simulink model "BLDCmotor_FOC_R2017b_fixdt"  (R2025a)
settings: Solver=FixedStepDiscrete  StartTime=0  StopTime=0.5  FixedStep=Ts  MaxStep=1e-6  RelTol=1e-6  AbsTol=1e-6  EnableMultiTasking=on
PreLoadFcn:
  | addpath(pwd);
  | addpath(genpath('01_Libraries'));
  | addpath(genpath('02_Figures'));
  | addpath(genpath('03_CreateParamTable'));
InitFcn:
  | init_model;
values from neighbouring files (symbols this model uses):
  a_cpr = 65535    [init_model.m]
  a_elecAngle = 60    [init_model.m]
  a_elecoffset = a_elecPeriod/12    (= 30)    [init_model.m]
  a_elecPeriod = 360    [init_model.m]
  a_fcpr = 1/65535    (= 1.52590218967e-05)    [init_model.m]
  a_mechoffset = a_elecoffset/n_polePairs    (= 5)    [init_model.m]
  a_phaAdvMax = 25    [init_model.m]
  b_angleMeasEna = 1    [init_model.m]
  b_cruiseCtrlEna = 0    [init_model.m]
  b_diagEna = 0    [init_model.m]
  b_fieldWeakEna = 0    [init_model.m]
  cf_currFilt = 0.692    [init_model.m]
  cf_idKi = Ki / (f_ctrl)    (= 0.00409061543436)    [init_model.m]
  cf_idKp = Kp    (= 0.0523598775598)    [init_model.m]
  cf_iqKi = Ki / (f_ctrl)    (= 0.00409061543436)    [init_model.m]
  cf_iqKiLimProt = 60 / (f_ctrl)    (= 0.00375)    [init_model.m]
  cf_iqKp = Kp    (= 0.0523598775598)    [init_model.m]
  cf_KbLimProt = Simulink.Parameter    [init_model.m]
  cf_nKi = 20.4 / (f_ctrl)    (= 0.001275)    [init_model.m]
  cf_nKiLimProt = 20 / (f_ctrl)    (= 0.00125)    [init_model.m]
  cf_nKp = 1.18    [init_model.m]
  cf_speedCoef = round(f_ctrl * a_mechAngle * (pi/180) * (30/pi))    [init_model.m]
  CTRL_FOC = 2    [init_model.m]
  CTRL_SIN = 1    [init_model.m]
  dV_openRate = 1000 / (f_ctrl)    (= 0.0625)    [init_model.m]
  dz_cntTrnsDetHi = 40    [init_model.m]
  dz_cntTrnsDetLo = 20    [init_model.m]
  ff_gain = ((r_motn / i_sca) * ((GD32_Vd_max_margin) / v_bus))    (= 0.338958333333)    [init_model.m]
  GD32_Vd_max_margin = GD32_Vd_max - V_margin    (= 1627)    [init_model.m]
  GD32_Vq_max_M1 = sqrt(GD32_Vd_max_margin^2 - GD32_Vq_max_XA.^2)    [init_model.m]
  i_max = i_max * i_sca    (= 500)    [init_model.m]
  id_fieldWeakMax = 5 * i_sca    (= 250)    [init_model.m]
  iq_maxSca_M1 = sqrt(1 - iq_maxSca_XA.^2)    [init_model.m]
  mcu_model = GD32F103    (= 1)    [init_model.m]
  n_commAcvLo = 15    [init_model.m]
  n_commDeacvHi = 30    [init_model.m]
  n_cruiseMotTgt = 0    [init_model.m]
  n_fieldWeakAuthHi = 300    [init_model.m]
  n_fieldWeakAuthLo = 100    [init_model.m]
  n_max = 1950    [init_model.m]
  n_polePairs = 6    [init_model.m]
  n_stdStillDet = 3    [init_model.m]
  OPEN_MODE = 0    [init_model.m]
  r_cos_M1 = cos((a_elecAngle_XA + a_elecPeriod/12)*(pi/180))    [init_model.m]
  r_errInpTgtThres = 600    [init_model.m]
  r_fieldWeakHi = 1000    [init_model.m]
  r_fieldWeakLo = 750    [init_model.m]
  r_motn = r_mot/2    (= 0.25)    [init_model.m]
  r_sin3PhaA_M1 = sin3Arm + A*r_sinPhaA_M1    [init_model.m]
  r_sin3PhaB_M1 = sin3Arm + A*r_sinPhaB_M1    [init_model.m]
  r_sin3PhaC_M1 = sin3Arm + A*r_sinPhaC_M1    [init_model.m]
  r_sin_M1 = sin((a_elecAngle_XA + a_elecPeriod/12)*(pi/180))    [init_model.m]
  SPD_MODE = 2    [init_model.m]
  STM32_Vd_max_margin = STM32_Vd_max - V_margin    (= 940)    [init_model.m]
  STM32_Vq_max_M1 = sqrt(STM32_Vd_max_margin^2 - STM32_Vq_max_XA.^2)    [init_model.m]
  t_errDequal = 1.80 * f_ctrl    (= 28800)    [init_model.m]
  t_errQual = 0.24 * f_ctrl    (= 3840)    [init_model.m]
  tgt_scale = 2047    [init_model.m]
  TRQ_MODE = 3    [init_model.m]
  Ts = 5e-6    (= 5e-06)    [init_model.m]
  Ts_ctrl = 6e-5    (= 6e-05)    [init_model.m]
  v_bus = 24    [init_model.m]
  vec_hallToPos = [0 2 0 1 4 3 5 0]    [init_model.m]
  VLT_MODE = 1    [init_model.m]
  z_commutMap_M1 = [-1 -1  0  1  1  0 ... (first row only)    [init_model.m]
  z_ctrlModReq = TRQ_MODE    (= 3)    [init_model.m]
  z_ctrlTypSel = CTRL_FOC    (= 2)    [init_model.m]
  z_maxCntRst = 2000    [init_model.m]
  z_selPhaCurMeasABC = 2    [init_model.m]
undefined symbols (not defined in the file or in its folder): BLDCmotor_FOC_R2017b_fixdt, DiscIntNeverNeededParam, DWORK0, DWORK1, DWORK2, DWORK3, powergui, spspowerguiLib
libraries: BLDC_controller_Lib x18, simulink x13, prociolib x6, eePwmGenerator x6, eePwmGeneratorMultilevel x3, mcbpositiondecoderlib x2, slpidlib x2, spsControlledVoltageSourceLib x1, spsMultimeterLib x1, spsPermanentMagnetSynchronousMachineLib x1, spsUniversalBridgeLib x1, spsVoltageMeasurementLib x1
(part 2 of 6)

== system BLDCmotor_FOC_R2017b_fixdt/PWM_gates ==
  DC_pha : Inport
  Abs : Abs  Commented=on  OutDataTypeStr=Inherit: Inherit via back propagation  RndMeth=Zero  SaturateOnIntegerOverflow=off
  Abs1 : Abs  Commented=on  OutDataTypeStr=Inherit: Inherit via back propagation  RndMeth=Zero  SaturateOnIntegerOverflow=off
  Abs2 : Abs  Commented=on  OutDataTypeStr=Inherit: Inherit via back propagation  RndMeth=Zero  SaturateOnIntegerOverflow=off
  Constant3 : Constant  Commented=on  Value=0  OutDataTypeStr=Inherit: Inherit via back propagation
  Constant4 : Constant  Commented=on  OutDataTypeStr=Inherit: Inherit via back propagation
  Demux : Demux  Commented=on  Outputs=3
  Demux1 : Demux  Commented=on  Outputs=3
  MCU_VD_Selector : Subsystem  Commented=on
  MinMax : MinMax  Commented=on  Inputs=2  OutDataTypeStr=Inherit: Inherit via back propagation  RndMeth=Zero
  MinMax1 : MinMax  Commented=on  Function=max  Inputs=2  OutDataTypeStr=Inherit: Inherit via back propagation  RndMeth=Zero
  MinMax2 : MinMax  Commented=on  Inputs=2  OutDataTypeStr=Inherit: Inherit via back propagation  RndMeth=Zero
  MinMax3 : MinMax  Commented=on  Function=max  Inputs=2  OutDataTypeStr=Inherit: Inherit via back propagation  RndMeth=Zero
  MinMax4 : MinMax  Commented=on  Inputs=2  OutDataTypeStr=Inherit: Inherit via back propagation  RndMeth=Zero
  MinMax5 : MinMax  Commented=on  Function=max  Inputs=2  OutDataTypeStr=Inherit: Inherit via back propagation  RndMeth=Zero
  Mux1 : Mux  Commented=on  Inputs=6
  Mux4 : Mux  Commented=on  Inputs=3
  "PWM Gate Signal Generator (Three-phase, Two-level)" : eePwmGeneratorTwoLevel/PWM Gate Signal Generator (Three-phase, Two-level)  Commented=on  fsw=1e3  Ts=5e-5
      settings: SamplingMode=Natural
      settings: LibrarySourceBlock=|
      | ee_sl_lib/Pulse Width
      | Modulation/PWM Gate Signal Generator
      | (Three-phase, Two-level)
  PWM Generator (2-Level) : spsPWMGenerator2LevelLib/PWM Generator (2-Level)  ModulatorType=Three-phase bridge (6 pulses)  ModulatorMode=Unsynchronized  Fc=16000  Pc=90  nF=27  MinMax=[-1627 1627]  SamplingTechnique=Natural  ModulatingSignals=off  m=0.8  Freq=60  Phase=0  Ts=Ts  ShowCarrierOutport=on
  PWM Generator (Multilevel) : eePwmGeneratorMultilevel/PWM Generator (Multilevel)  Commented=on  topology=Half-bridge  Nsm=1  Tper=6.25e-5  Ts=5e-6
      settings: LibrarySourceBlock=|
      | ee_sl_lib/Pulse Width
      | Modulation/PWM Generator
      | (Multilevel)
  PWM Generator (Multilevel)1 : eePwmGeneratorMultilevel/PWM Generator (Multilevel)  Commented=on  topology=Half-bridge  Nsm=1  Tper=6.25e-5  Ts=5e-6
      settings: LibrarySourceBlock=|
      | ee_sl_lib/Pulse Width
      | Modulation/PWM Generator
      | (Multilevel)
  PWM Generator (Multilevel)2 : eePwmGeneratorMultilevel/PWM Generator (Multilevel)  Commented=on  topology=Half-bridge  Nsm=1  Tper=6.25e-5  Ts=5e-6
      settings: LibrarySourceBlock=|
      | ee_sl_lib/Pulse Width
      | Modulation/PWM Generator
      | (Multilevel)
  PWM Write : prociolib/PWM Write  Commented=on  ShowPeriodInp=off  ShowPhaseInp=off  PeripheralConfigBtnCtrl=0  BlockSID=BLDCmotor_FOC_R2017b_fixdt:22845
  PWM Write1 : prociolib/PWM Write  Commented=on  ShowPeriodInp=off  ShowPhaseInp=off  PeripheralConfigBtnCtrl=0  BlockSID=BLDCmotor_FOC_R2017b_fixdt:22846
  PWM Write2 : prociolib/PWM Write  Commented=on  ShowPeriodInp=off  ShowPhaseInp=off  PeripheralConfigBtnCtrl=0  BlockSID=BLDCmotor_FOC_R2017b_fixdt:22847
  PWM Write3 : prociolib/PWM Write  Commented=on  ShowPeriodInp=off  ShowPhaseInp=off  PeripheralConfigBtnCtrl=0  BlockSID=BLDCmotor_FOC_R2017b_fixdt:22848
  PWM Write4 : prociolib/PWM Write  Commented=on  ShowPeriodInp=off  ShowPhaseInp=off  PeripheralConfigBtnCtrl=0  BlockSID=BLDCmotor_FOC_R2017b_fixdt:22849
  PWM Write5 : prociolib/PWM Write  Commented=on  ShowPeriodInp=off  ShowPhaseInp=off  PeripheralConfigBtnCtrl=0  BlockSID=BLDCmotor_FOC_R2017b_fixdt:22850
  PWM_generator{,6..10} (6 alike) : eePwmGenerator/PWM Generator  Commented=on  CarrCount=Up  Tper=5e-05  Tdelay=0  Ts=Ts
  PWM_generator1 : Subsystem  Commented=on
      mask help: Simulink:masks:GenSFuncDesc_MD
      mask Help: eval('feval(''rtwprivate'',''rtwhelpview'',''rtw_sfcn_block'')');
  PWM_generator12 : Subsystem  Commented=on
      mask help: Simulink:masks:GenSFuncDesc_MD
      mask Help: eval('feval(''rtwprivate'',''rtwhelpview'',''rtw_sfcn_block'')');
  PWM_generator2 : Subsystem  Commented=on
      mask help: Simulink:masks:GenSFuncDesc_MD
      mask Help: eval('feval(''rtwprivate'',''rtwhelpview'',''rtw_sfcn_block'')');
  PWM_generator3 : Subsystem  Commented=on
      mask help: Simulink:masks:GenSFuncDesc_MD
      mask Help: eval('feval(''rtwprivate'',''rtwhelpview'',''rtw_sfcn_block'')');
  PWM_generator4 : Subsystem  Commented=on
      mask help: Simulink:masks:GenSFuncDesc_MD
      mask Help: eval('feval(''rtwprivate'',''rtwhelpview'',''rtw_sfcn_block'')');
  PWM_generator5 : Subsystem  Commented=on
      mask help: Simulink:masks:GenSFuncDesc_MD
      mask Help: eval('feval(''rtwprivate'',''rtwhelpview'',''rtw_sfcn_block'')');
  Terminator : Terminator
  Vd_max2 : Constant  Commented=on  Value=mcu_model  OutDataTypeStr=boolean
  signal_log6 : Subsystem  Commented=on
  gates_PWM : Outport  VectorParamsAs1DForOutWhenUnconnected=off
  wires:
  MCU_VD_Selector/1(Out1) -> ?
  Vd_max2/1 -> MCU_VD_Selector/1(In1)
  PWM Generator (Multilevel)1/1 -> Mux4/2
  Demux/3 -> PWM Generator (Multilevel)2/1
  Demux/2 -> PWM Generator (Multilevel)1/1
  ? -> Demux/1
  PWM Generator (Multilevel)/1 -> Mux4/1
  Demux/1 -> PWM Generator (Multilevel)/1
  PWM Generator (Multilevel)2/1 -> Mux4/3
  Abs2/1 -> PWM_generator10/1
  MinMax3/1 -> PWM_generator7/1
  PWM_generator8/1 -> Mux1/4
  MinMax5/1 -> PWM_generator9/1
  Abs1/1 -> PWM_generator8/1
  MinMax2/1 -> Abs1/1
  MinMax4/1 -> Abs2/1
  Abs/1 -> PWM_generator6/1
  PWM_generator6/1 -> Mux1/2
  Demux1/1 -> MinMax/2, MinMax1/2
  PWM_generator7/1 -> Mux1/3
  MinMax/1 -> Abs/1
  Demux1/2 -> MinMax2/2, MinMax3/2
  PWM_generator/1 -> Mux1/1
  PWM_generator9/1 -> Mux1/5
  Constant4/1 -> MinMax5/1, MinMax3/1, MinMax1/1
  MinMax1/1 -> PWM_generator/1
  PWM_generator10/1 -> Mux1/6
  Demux1/3 -> MinMax5/2, MinMax4/2
  Constant3/1 -> MinMax4/1, MinMax2/1, MinMax/1
  ? -> Demux1/1
  DC_pha/1 -> PWM Generator (2-Level)/1
  PWM Generator (2-Level)/1 -> gates_PWM/1
  PWM Generator (2-Level)/2 -> Terminator/1

== system BLDCmotor_FOC_R2017b_fixdt/Power Stage ==
  DC_pha : Inport
  LdTrq : Inport  Port=2
  Bus Creator : BusCreator  Inputs=4
  Bus Creator1 : BusCreator  Inputs=13
  Bus Selector : BusSelector  OutputSignals=signal1.IaStator,signal1.IbStator,signal1.IcStator,signal1.IqSync,signal1.IdSync,signal1.VqSync,signal1.VdSync,Hall.signal1,Hall.signal2,Hall.signal3  OutputAsBus=on
  Bus Selector1 : BusSelector  OutputSignals=signal1.MtrSpd,signal1.MtrPos,signal1.MtrTrq  OutputAsBus=on
  Bus Selector3 : BusSelector  OutputSignals=MtrElcPos  OutputAsBus=on
  Constant1 : Constant  Value=v_bus
  Data Type Conversion9 : DataTypeConversion  OutDataTypeStr=double  SaturateOnIntegerOverflow=off
  Demux1 : Demux  Outputs=[1,1,1,1,1,1,1,1,1,1]
  Demux2 : Demux  Outputs=[1,1,1]
  Divide : Product  Inputs=*/
  Product : Product
  Scope : Scope  NumInputPorts=3
      settings: ActiveDisplayYMinimum=-159.83844430308204  ActiveDisplayYMaximum=171.67027137436321  DataLoggingVariableName=ScopeData12
  Subsystem : Subsystem
  Surface Mount PMSM : autolibpmsmexterior/Surface Mount PMSM  port_config=Torque  sim_type=Discrete  Ts=5e-06  P=n_polePairs  Rs=r_motn  Ldq_=L_ph  KConstText=Torque constant (Kt):  lambda_pm=0.2205  Ke=160  Kt=1  mechanical=[0.0027, 0.1, 0]  idq0=[0 0]  theta_init=0  omega_init=0  KConst=0.2205  lambda_pm_calc=0.2205  RefBlkName='autolibpmsmexterior/Surface Mount PMSM'  aMode=5  Ldq="[0.0017      0.0017]"
  Variant Subsystem : Subsystem  Variant=on  VariantActivationTime=code compile
  motor_out : Outport  VectorParamsAs1DForOutWhenUnconnected=off
  wires:
  Data Type Conversion9/1 -> Divide/2
  Variant Subsystem/1(Vd_max_margin) -> Data Type Conversion9/1
  DC_pha/1 -> Scope/3, Product/2
  Product/1 -> Scope/2, Surface Mount PMSM/2
  Surface Mount PMSM/2 -> Bus Creator/2
  Surface Mount PMSM/3 -> Bus Creator/3
  LdTrq/1 -> Surface Mount PMSM/1
  Bus Creator/1 -> Bus Selector/1, Bus Selector1/1
  Bus Creator1/1 -> motor_out/1  "<IcStator>"
  Bus Selector3/1 -> Subsystem/1(the)
  Surface Mount PMSM/1 -> Bus Selector3/1, Bus Creator/1
  Demux1/1 -> Bus Creator1/1  "Stator current is_a (A)"
  Demux1/8 -> Bus Creator1/8  "Hall effect signal h_a"
  Demux1/10 -> Bus Creator1/10  "Hall effect signal h_c"
  Demux2/1 -> Bus Creator1/11  "Rotor speed wm (rad/s)"
  Demux2/3 -> Bus Creator1/13  "Electromagnetic torque Te (N*m)"
  Demux1/6 -> Bus Creator1/6  "Stator voltage Vs_q (V)"
  Demux1/9 -> Bus Creator1/9  "Hall effect signal h_b"
  Demux1/2 -> Bus Creator1/2  "Stator current is_b (A)"
  Demux1/5 -> Bus Creator1/5  "Stator current is_d (A)"
  Demux1/4 -> Bus Creator1/4  "Stator current is_q (A)"
  Demux1/7 -> Bus Creator1/7  "Stator voltage Vs_d (V)"
  Demux1/3 -> Bus Creator1/3  "Stator current is_c (A)"
  Demux2/2 -> Bus Creator1/12  "Rotor angle thetam (rad)"
  Subsystem/1(Hall) -> Bus Creator/4  "Hall"
  Bus Selector/1 -> Demux1/1
  Bus Selector1/1 -> Demux2/1
  Constant1/1 -> Divide/1
  Divide/1 -> Scope/1, Product/1

== system BLDCmotor_FOC_R2017b_fixdt/Theoretical_Speed_Trajectory ==
  note: Ideal Speed Trajectory Calculation
      | Based on Min/Max torque and Min/Max torque rate constraints
  r_inpTgtRaw : Inport
  Discrete Derivative1 : simulink/Discrete/Discrete Derivative  gainval=1.0  ICPrevScaledInput=0.0  OutMin=[]  OutMax=[]  OutDataType=fixdt(1, 16)  OutScaling=2^-10  DoSatur=off
  Discrete Derivative2 : simulink/Discrete/Discrete Derivative  gainval=1.0  ICPrevScaledInput=0.0  OutMin=[]  OutMax=[]  OutDataType=fixdt(1, 16)  OutScaling=2^-10  DoSatur=off
  Discrete-Time Integrator2 : DiscreteIntegrator  SampleTime=-1  ICPrevOutput=DiscIntNeverNeededParam  ICPrevScaledInput=DiscIntNeverNeededParam
  Divide2 : Product  Inputs=*/
  Divide3 : Product  Inputs=**
  Divide4 : Product  Inputs=**
  Gain1 : Gain  Gain=-1
  Gain2 : Gain  Gain=-1
  Gain4 : Gain  Gain=pi/30
  Gain5 : Gain  Gain=30/pi
  J_mot : Constant  Value=0.01  OutDataTypeStr=Inherit: Inherit via back propagation
  Kp : Constant  Value=65  OutDataTypeStr=Inherit: Inherit via back propagation
  M_max : Constant  Value=15  OutDataTypeStr=Inherit: Inherit via back propagation
  Manual Switch : ManualSwitch
  Mux4 : Mux  Inputs=2
  Rate Limiter Dynamic3 : simulink/Discontinuities/Rate Limiter Dynamic
  Saturation Dynamic : simulink/Discontinuities/Saturation Dynamic  OutMin=[]  OutMax=[]  OutDataTypeStr=Inherit: Same as second input  OutDataType=fixdt(1, 16)  OutScaling=2^-10  DoSatur=off
  Scope : Scope  NumInputPorts=3
      settings: ActiveDisplayYMinimum=-1250  ActiveDisplayYMaximum=1250
  Sum2 : Sum  Inputs=|+-  RndMeth=Zero  OutDataTypeStr=Inherit: Same as first input
  Sum8 : Sum  Inputs=++|  RndMeth=Zero  OutDataTypeStr=Inherit: Same as first input
  dM_max : Constant  Value=500  OutDataTypeStr=Inherit: Inherit via back propagation
  r_inpTgt : Outport  VectorParamsAs1DForOutWhenUnconnected=off
  wires:
  Gain4/1 -> Divide4/2  "dw"
  M_max/1 -> Gain1/1, Saturation Dynamic/1
  J_mot/1 -> Divide2/2, Divide4/1
  Divide2/1 -> Gain5/1  "w"
  [r_inpTgtRaw] -> Discrete Derivative2/1, Sum2/1
  Divide4/1 -> Saturation Dynamic/2  "M"
  Gain1/1 -> Saturation Dynamic/3
  dM_max/1 -> Gain2/1, Rate Limiter Dynamic3/1
  Sum2/1 -> Divide3/2
  Divide3/1 -> Sum8/2
  Rate Limiter Dynamic3/1 -> [M_tgtTheo], Discrete-Time Integrator2/1
  Gain2/1 -> Rate Limiter Dynamic3/3
  Sum8/1 -> Gain4/1  "dn"
  Saturation Dynamic/1 -> Rate Limiter Dynamic3/2
  Gain5/1 -> [r_inpTgt], Sum2/2  "rpm"
  Kp/1 -> Divide3/1
  Discrete-Time Integrator2/1 -> Divide2/1
  Mux4/1 -> Scope/1
  Discrete Derivative1/1 -> Scope/3
  Discrete Derivative2/1 -> Sum8/1
  [M_tgtTheo] -> Discrete Derivative1/1, Scope/2
  r_inpTgtRaw/1 -> [r_inpTgtRaw]
  [r_inpTgtRaw] -> Mux4/1
  [r_inpTgt] -> Mux4/2
  [r_inpTgt] -> Manual Switch/2
  Manual Switch/1 -> r_inpTgt/1
  [r_inpTgtRaw] -> Manual Switch/1

== system BLDCmotor_FOC_R2017b_fixdt/filtLowPass ==
  u : Inport
  coef : Inport  Port=2
  Data Type Conversion23 : DataTypeConversion  OutDataTypeStr=fixdt(1,32,6)  SaturateOnIntegerOverflow=off  RndMeth=Floor
  Low_Pass_Filter : Subsystem
      settings: RTWFcnNameOpts=Use subsystem name
      mask Display:
      | plot(0,0,100,100, ...
      | [73,75,73,75,25,25,28,25,22,25],[18,20,22,20,20,84,82,84,82,84], ...
      | [25,33,33,72],[20,20,70,70],[33,34,36,39,44,50,56,66,73],[20,25,33,43,55,63,66,70,70]);
      | text(50,40,'coef'),
  y : Outport  VectorParamsAs1DForOutWhenUnconnected=off
  wires:
  coef/1 -> Low_Pass_Filter/2(coef)
  Low_Pass_Filter/1(y) -> y/1
  u/1 -> Data Type Conversion23/1
  Data Type Conversion23/1 -> Low_Pass_Filter/1(u)

== system BLDCmotor_FOC_R2017b_fixdt/mixer ==
  speed : Inport
  steer : Inport  Port=2
  speed_coef : Inport  Port=3
  steer_coef : Inport  Port=4
  Data Type Conversion2 : DataTypeConversion  OutDataTypeStr=int16  SaturateOnIntegerOverflow=off  RndMeth=Floor
  Data Type Conversion3 : DataTypeConversion  OutDataTypeStr=int16  SaturateOnIntegerOverflow=off  RndMeth=Floor
  Data Type Conversion4 : DataTypeConversion  OutDataTypeStr=int16  SaturateOnIntegerOverflow=off  RndMeth=Floor
  Display : Display
  Display1 : Display
  Display3 : Display
  Divide1 : Product  Inputs=**  RndMeth=Simplest  OutDataTypeStr=Inherit: Same as first input
  Divide2 : Product  Inputs=**  RndMeth=Simplest  OutDataTypeStr=Inherit: Same as first input
  Sum1 : Sum  Inputs=+-  InputSameDT=on  RndMeth=Simplest  SaturateOnIntegerOverflow=on  OutDataTypeStr=Inherit: Same as first input
  Sum2 : Sum  InputSameDT=on  RndMeth=Simplest  SaturateOnIntegerOverflow=on  OutDataTypeStr=Inherit: Same as first input
  speedR : Outport  VectorParamsAs1DForOutWhenUnconnected=off
  speedL : Outport  Port=2  VectorParamsAs1DForOutWhenUnconnected=off
  wires:
  Sum1/1 -> Data Type Conversion2/1
  speed/1 -> [speed]
  steer/1 -> [steer]
  speed_coef/1 -> [speed_coef]
  steer_coef/1 -> [steer_coef]
  [speed] -> Divide1/1
  [speed_coef] -> Divide1/2
  [steer] -> Divide2/1
  [steer_coef] -> Divide2/2
  Divide1/1 -> Display1/1, Data Type Conversion4/1, Sum2/1, Sum1/1
  Divide2/1 -> Sum2/2, Sum1/2
  Data Type Conversion2/1 -> speedR/1
  Data Type Conversion3/1 -> speedL/1
  Data Type Conversion4/1 -> Display/1
  Sum2/1 -> Display3/1, Data Type Conversion3/1

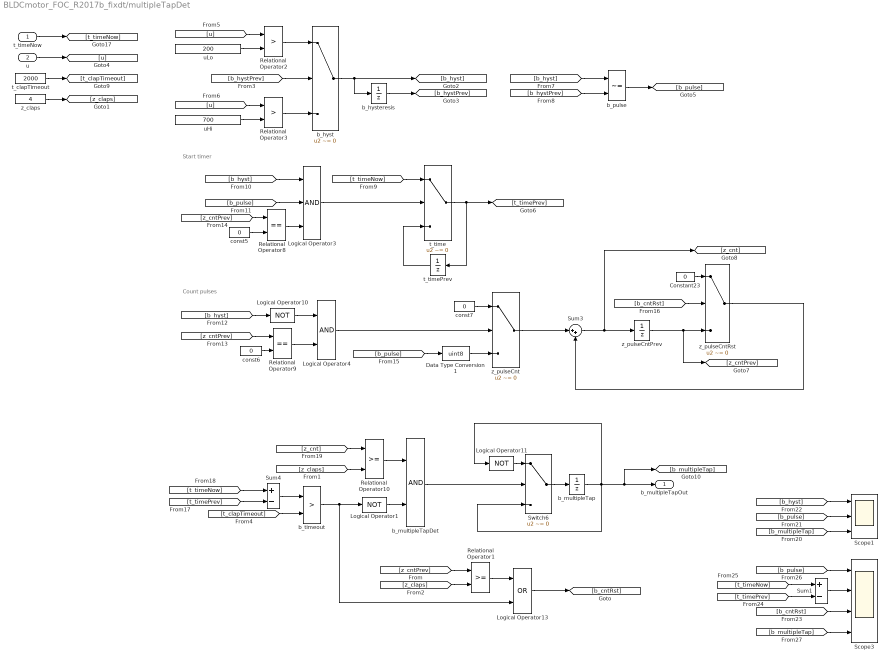
== system BLDCmotor_FOC_R2017b_fixdt/multipleTapDet ==
  note: Count pulses
  note: Start timer
  t_timeNow : Inport
  u : Inport  Port=2
  Constant23 : Constant  Value=0  OutDataTypeStr=Inherit: Inherit via back propagation
  Data Type Conversion1 : DataTypeConversion  OutDataTypeStr=uint8  SaturateOnIntegerOverflow=off  RndMeth=Floor
  Logical Operator1 : Logic  Operator=NOT  AllPortsSameDT=off  OutDataTypeStr=boolean
  Logical Operator10 : Logic  Operator=NOT  AllPortsSameDT=off  OutDataTypeStr=boolean
  Logical Operator11 : Logic  Operator=NOT  AllPortsSameDT=off  OutDataTypeStr=boolean
  Logical Operator13 : Logic  Operator=OR  AllPortsSameDT=off  OutDataTypeStr=boolean
  Logical Operator3 : Logic  Inputs=3  AllPortsSameDT=off  OutDataTypeStr=boolean
  Logical Operator4 : Logic  AllPortsSameDT=off  OutDataTypeStr=boolean
  Relational Operator1 : RelationalOperator  OutDataTypeStr=boolean  RndMeth=Simplest  InputSameDT=off
  Relational Operator10 : RelationalOperator  OutDataTypeStr=boolean  RndMeth=Simplest  InputSameDT=off
  Relational Operator2 : RelationalOperator  Operator=>  OutDataTypeStr=boolean  RndMeth=Simplest  InputSameDT=off
  Relational Operator3 : RelationalOperator  Operator=>  OutDataTypeStr=boolean  RndMeth=Simplest  InputSameDT=off
  Relational Operator8 : RelationalOperator  Operator===  OutDataTypeStr=boolean  RndMeth=Simplest  InputSameDT=off
  Relational Operator9 : RelationalOperator  Operator===  OutDataTypeStr=boolean  RndMeth=Simplest  InputSameDT=off
  Scope1 : Scope  NumInputPorts=3
      settings: ActiveDisplayYMinimum=-0.125  ActiveDisplayYMaximum=1.125
  Scope3 : Scope  NumInputPorts=4
      settings: ActiveDisplayYMinimum=-0.125  ActiveDisplayYMaximum=1.125
  Sum1 : Sum  Inputs=+-
  Sum3 : Sum  Inputs=|++
  Sum4 : Sum  Inputs=+-
  Switch6 : Switch  Criteria=u2 ~= 0  OutDataTypeStr=Inherit: Inherit via back propagation  RndMeth=Zero  SaturateOnIntegerOverflow=off  InputSameDT=off
  b_hyst : Switch  Criteria=u2 ~= 0  RndMeth=Zero  SaturateOnIntegerOverflow=off  InputSameDT=off
  b_hysteresis : UnitDelay  SampleTime=-1  HasFrameUpgradeWarning=on
      settings: AttributesFormatString=Ini=%<X0>
  b_multipleTap : UnitDelay  SampleTime=-1  HasFrameUpgradeWarning=on
      settings: AttributesFormatString=Ini=%<X0>
  b_multipleTapDet : Logic  AllPortsSameDT=off  OutDataTypeStr=boolean
  b_pulse : RelationalOperator  Operator=~=  OutDataTypeStr=boolean  RndMeth=Simplest  InputSameDT=off
  b_timeout : RelationalOperator  Operator=>  OutDataTypeStr=boolean  RndMeth=Simplest  InputSameDT=off
  const5 : Constant  Value=0  OutDataTypeStr=Inherit: Inherit via back propagation
  const6 : Constant  Value=0  OutDataTypeStr=Inherit: Inherit via back propagation
  const7 : Constant  Value=0  OutDataTypeStr=Inherit: Inherit via back propagation
  t_clapTimeout : Constant  Value=2000  OutDataTypeStr=Inherit: Inherit via back propagation
  t_time : Switch  Criteria=u2 ~= 0  OutDataTypeStr=Inherit: Inherit via back propagation  RndMeth=Zero  SaturateOnIntegerOverflow=off  InputSameDT=off
  t_timePrev : UnitDelay  SampleTime=-1  HasFrameUpgradeWarning=on
      settings: AttributesFormatString=Ini=%<X0>
  uHi : Constant  Value=700  OutDataTypeStr=Inherit: Inherit via back propagation
  uLo : Constant  Value=200  OutDataTypeStr=Inherit: Inherit via back propagation
  z_claps : Constant  Value=4  OutDataTypeStr=Inherit: Inherit via back propagation
  z_pulseCnt : Switch  Criteria=u2 ~= 0  OutDataTypeStr=Inherit: Inherit via back propagation  RndMeth=Zero  SaturateOnIntegerOverflow=off  InputSameDT=off
  z_pulseCntPrev : UnitDelay  SampleTime=-1  HasFrameUpgradeWarning=on
      settings: AttributesFormatString=Ini=%<X0>
  z_pulseCntRst : Switch  Criteria=u2 ~= 0  OutDataTypeStr=Inherit: Inherit via back propagation  RndMeth=Simplest  SaturateOnIntegerOverflow=off  InputSameDT=off
  b_multipleTapOut : Outport  VectorParamsAs1DForOutWhenUnconnected=off
  wires:
  t_timeNow/1 -> [t_timeNow]
  Relational Operator2/1 -> b_hyst/1
  b_hyst/1 -> b_hysteresis/1, [b_hyst]
  uLo/1 -> Relational Operator2/2
  b_hysteresis/1 -> [b_hystPrev]
  [b_hystPrev] -> b_hyst/2
  uHi/1 -> Relational Operator3/2
  Relational Operator3/1 -> b_hyst/3
  u/1 -> [u]
  [u] -> Relational Operator2/1
  [u] -> Relational Operator3/1
  [b_hyst] -> b_pulse/1
  [b_hystPrev] -> b_pulse/2
  b_pulse/1 -> [b_pulse]
  t_time/1 -> t_timePrev/1, [t_timePrev]
  t_timePrev/1 -> t_time/3
  [t_timeNow] -> t_time/1
  const5/1 -> Relational Operator8/2
  Relational Operator8/1 -> Logical Operator3/3
  Logical Operator3/1 -> t_time/2
  [b_hyst] -> Logical Operator3/1
  [b_pulse] -> Logical Operator3/2
  Data Type Conversion1/1 -> z_pulseCnt/3
  const7/1 -> z_pulseCnt/1
  Logical Operator4/1 -> z_pulseCnt/2
  const6/1 -> Relational Operator9/2
  Relational Operator9/1 -> Logical Operator4/2
  Logical Operator10/1 -> Logical Operator4/1
  [b_pulse] -> Data Type Conversion1/1
  [b_hyst] -> Logical Operator10/1
  [z_cntPrev] -> Relational Operator9/1
  [z_cntPrev] -> Relational Operator8/1
  z_pulseCnt/1 -> Sum3/1
  Sum4/1 -> b_timeout/1
  [t_timePrev] -> Sum4/2
  [t_timeNow] -> Sum4/1
  [t_clapTimeout] -> b_timeout/2
  Logical Operator11/1 -> Switch6/1
  b_multipleTap/1 -> Switch6/3, [b_multipleTap], b_multipleTapOut/1, Logical Operator11/1
  Switch6/1 -> b_multipleTap/1
  [z_claps] -> Relational Operator10/2
  [z_cnt] -> Relational Operator10/1
  Relational Operator10/1 -> b_multipleTapDet/1
  b_timeout/1 -> Logical Operator13/2, Logical Operator1/1
  [b_pulse] -> Scope1/2
  [b_hyst] -> Scope1/1
  b_multipleTapDet/1 -> Switch6/2
  Logical Operator13/1 -> [b_cntRst]
  [z_cntPrev] -> Relational Operator1/1
  [z_claps] -> Relational Operator1/2
  Relational Operator1/1 -> Logical Operator13/1
  [b_cntRst] -> z_pulseCntRst/2
  Constant23/1 -> z_pulseCntRst/1
  z_pulseCntPrev/1 -> [z_cntPrev], z_pulseCntRst/3
  z_pulseCntRst/1 -> Sum3/2
  z_claps/1 -> [z_claps]
  t_clapTimeout/1 -> [t_clapTimeout]
  Logical Operator1/1 -> b_multipleTapDet/2
  Sum3/1 -> [z_cnt], z_pulseCntPrev/1
  [t_timeNow] -> Sum1/1
  [t_timePrev] -> Sum1/2
  [b_pulse] -> Scope3/1
  Sum1/1 -> Scope3/2
  [b_cntRst] -> Scope3/3
  [b_multipleTap] -> Scope1/3
  [b_multipleTap] -> Scope3/4

== system BLDCmotor_FOC_R2017b_fixdt/rad2deg ==
  note: Convert mechanical angle to electrical angle.
  rad : Inport
  Constant : Constant  Value=360
  Constant1 : Constant  Value=n_polePairs
  Divide : Product  Inputs=**
  Gain4 : Gain  Gain=180/pi  RndMeth=Zero  OutDataTypeStr=Inherit: Same as input
  Math Function : Math  Operator=mod  SignedPower=on
  deg : Outport  VectorParamsAs1DForOutWhenUnconnected=off
  wires:
  Math Function/1 -> deg/1
  rad/1 -> Gain4/1
  Constant/1 -> Math Function/2
  Gain4/1 -> Divide/1  "deg"
  Constant1/1 -> Divide/2
  Divide/1 -> Math Function/1

== system BLDCmotor_FOC_R2017b_fixdt/rad2deg1 ==
  rad : Inport
  Constant : Constant  Value=360
  Constant1 : Constant  Value=n_polePairs  OutDataTypeStr=uint8
  Constant2 : Constant  Value=360
  Constant3 : Constant  Commented=on  Value=360
  Divide : Product  Inputs=**
  Divide1 : Product  Commented=on  Inputs=*/
  Gain : Gain  Gain=a_cpr
  Gain1 : Gain  Gain=1/360
  Gain4 : Gain  Gain=180/pi  RndMeth=Zero  OutDataTypeStr=Inherit: Same as input
  Math Function : Math  Operator=mod  SignedPower=on
  Math Function1 : Math  Operator=mod  SignedPower=on
  Scope : Scope  NumInputPorts=3
      settings: PlotAsMagnitudePhase=on  ActiveDisplayYMinimum=11136.298351792939  ActiveDisplayYMaximum=38594.176596311016  DataLoggingVariableName=ScopeData2
  counts : Outport  VectorParamsAs1DForOutWhenUnconnected=off
  deg : Outport  Port=2  VectorParamsAs1DForOutWhenUnconnected=off
  wires:
  Constant/1 -> Math Function/2
  Constant1/1 -> Divide/2
  Constant2/1 -> Math Function1/2
  Divide/1 -> Math Function1/1
  Math Function1/1 -> Scope/3
  Gain4/1 -> Math Function/1
  rad/1 -> Gain4/1
  Constant3/1 -> Divide1/1
  Gain/1 -> Gain1/1
  Gain1/1 -> counts/1, Scope/1
  Math Function/1 -> Gain/1, Scope/2, deg/1, Divide/1

== system BLDCmotor_FOC_R2017b_fixdt/rateLimiter ==
  u : Inport
  rate : Inport  Port=2
  Data Type Conversion1 : DataTypeConversion  OutDataTypeStr=fixdt(1,16,6)  SaturateOnIntegerOverflow=off  RndMeth=Floor
  Gain : Gain  Tag=struct('comment',struct('text','','placement',1),'logdata',struct('maxnumvals',inf,'plotchannels',[],'loggingmode',3,'channels',1),'output',struct('variable','','description','','name','$S_$B','width',1,'address','','max',NaN,'min',NaN,'class','default','type','CONTINUOUS','scaling','','lsb',1,'offset',0,'arb',0,'freeze',1,'unit','','autoscalingmode',1,'lowerheadroom',1,'upperheadroom',1,'headroomunit','bit','keepdatatype',1,'checkmin',0,'checkmax',0,'castoutput',0,'show',0),'gain',struct('variable','','description','','name','$S_$B_gain','width',1,'address','','max',NaN,'min',NaN,'class','default','type','CONTINUOUS','scaling','','lsb',1,'offset',0,'arb',0,'freeze',1,'unit','','keepdatatype',1,'value','1','scalar',0,'tolerance',1),'scalingvalid',0,'date',730486)  Gain=-1  RndMeth=Zero  OutDataTypeStr=Inherit: Same as input  ParamDataTypeStr=Inherit: Same as input
  Rate_Limiter : Subsystem
      settings: RTWFcnNameOpts=Use subsystem name
      mask Display: plot([0.15 0.85],[0.5 0.5],[0.5 0.5],[0.1 0.9],[0.25 0.75],[0.1 0.9])
  y : Outport  VectorParamsAs1DForOutWhenUnconnected=off
  wires:
  Data Type Conversion1/1 -> Rate_Limiter/1(u)
  u/1 -> Data Type Conversion1/1
  Rate_Limiter/1(y) -> y/1
  rate/1 -> Gain/1, Rate_Limiter/2(inc)
  Gain/1 -> Rate_Limiter/3(dec)

== system BLDCmotor_FOC_R2017b_fixdt/shift ==
  note: Shift back by +30 deg due to angle calculation inside the controller.
  in : Inport
  Constant : Constant  Value=360
  Fcn8 : Fcn  Expr=u+30
  Math Function : Math  Operator=mod  SignedPower=on
  out : Outport  VectorParamsAs1DForOutWhenUnconnected=off
  wires:
  Constant/1 -> Math Function/2
  Math Function/1 -> out/1
  Fcn8/1 -> Math Function/1
  in/1 -> Fcn8/1

== system BLDCmotor_FOC_R2017b_fixdt/BLDC_controller/Call_Scheduler ==
  note: Call Squeduler : This creates a pulse train for task scheduling in series.
  Data Type Conversion : DataTypeConversion  OutDataTypeStr=boolean  SaturateOnIntegerOverflow=off  RndMeth=Floor
  Logical Operator2 : Logic  Commented=on  Operator=NOT  AllPortsSameDT=off  OutDataTypeStr=boolean
  UnitDelay2 : UnitDelay  InitialCondition=1  SampleTime=-1  HasFrameUpgradeWarning=on
      settings: AttributesFormatString=Ini=%<X0>
  UnitDelay4 : UnitDelay  Commented=on  InitialCondition=1  SampleTime=-1  HasFrameUpgradeWarning=on
      settings: AttributesFormatString=Ini=%<X0>
  UnitDelay5 : UnitDelay  SampleTime=-1  HasFrameUpgradeWarning=on
      settings: AttributesFormatString=Ini=%<X0>
  UnitDelay6 : UnitDelay  SampleTime=-1  HasFrameUpgradeWarning=on
      settings: AttributesFormatString=Ini=%<X0>
  call1 : Outport  OutputWhenDisabled=reset  InitialOutput=0  VectorParamsAs1DForOutWhenUnconnected=off
  call2 : Outport  Port=2  OutputWhenDisabled=reset  InitialOutput=0  VectorParamsAs1DForOutWhenUnconnected=off
  call3 : Outport  Port=3  OutputWhenDisabled=reset  InitialOutput=0  VectorParamsAs1DForOutWhenUnconnected=off
  wires:
  Logical Operator2/1 -> UnitDelay4/1
  UnitDelay4/1 -> Logical Operator2/1
  UnitDelay2/1 -> call1/1, UnitDelay5/1
  UnitDelay6/1 -> call3/1, Data Type Conversion/1
  UnitDelay5/1 -> call2/1, UnitDelay6/1
  Data Type Conversion/1 -> UnitDelay2/1

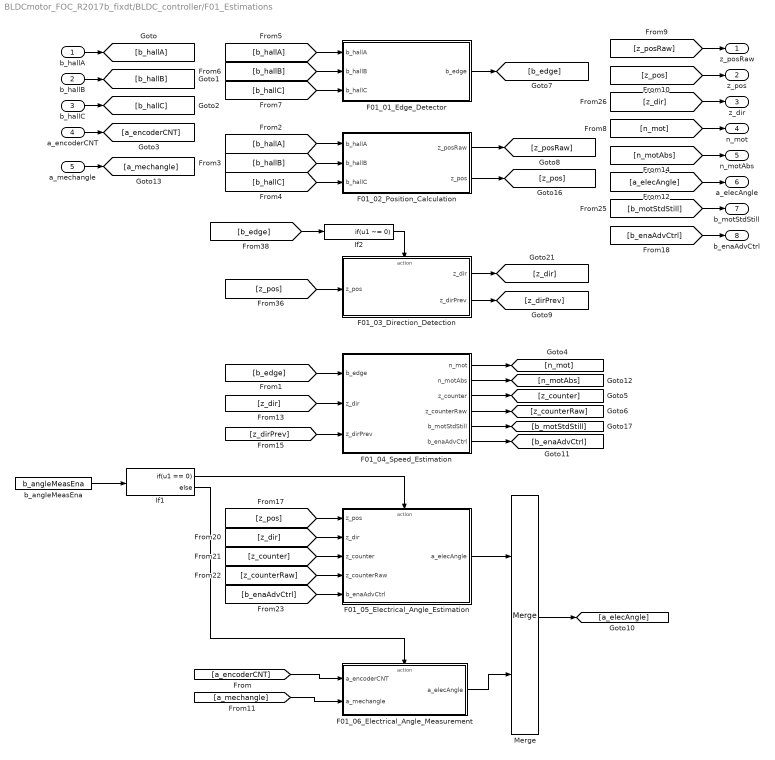
== system BLDCmotor_FOC_R2017b_fixdt/BLDC_controller/F01_Estimations ==
  b_hallA : Inport
  b_hallB : Inport  Port=2
  b_hallC : Inport  Port=3
  a_encoderCNT : Inport  Port=4
  a_mechangle : Inport  Port=5
  F01_01_Edge_Detector : Subsystem
  F01_02_Position_Calculation : Subsystem
  F01_03_Direction_Detection : Subsystem
  F01_04_Speed_Estimation : Subsystem
  F01_05_Electrical_Angle_Estimation : Subsystem
  F01_06_Electrical_Angle_Measurement : Subsystem
  If1 : If  IfExpression=u1 == 0
  If2 : If  IfExpression=u1 ~= 0  ShowElse=off
  Merge : Merge
  b_angleMeasEna : Constant  Value=b_angleMeasEna  OutDataTypeStr=boolean
  z_posRaw : Outport  OutputWhenDisabled=reset  InitialOutput=0  VectorParamsAs1DForOutWhenUnconnected=off
  z_pos : Outport  Port=2  OutputWhenDisabled=reset  InitialOutput=0  VectorParamsAs1DForOutWhenUnconnected=off
  z_dir : Outport  Port=3  OutputWhenDisabled=reset  InitialOutput=0  VectorParamsAs1DForOutWhenUnconnected=off
  "n_mot " : Outport  Port=4  OutputWhenDisabled=reset  InitialOutput=0  VectorParamsAs1DForOutWhenUnconnected=off
  n_motAbs : Outport  Port=5  OutputWhenDisabled=reset  InitialOutput=0  VectorParamsAs1DForOutWhenUnconnected=off
  a_elecAngle : Outport  Port=6  OutputWhenDisabled=reset  InitialOutput=0  VectorParamsAs1DForOutWhenUnconnected=off
  b_motStdStill : Outport  Port=7  OutputWhenDisabled=reset  InitialOutput=0  VectorParamsAs1DForOutWhenUnconnected=off
  b_enaAdvCtrl : Outport  Port=8  VectorParamsAs1DForOutWhenUnconnected=off
  wires:
  If2/1 -> F01_03_Direction_Detection/Action
  [b_edge] -> If2/1
  [z_pos] -> F01_03_Direction_Detection/1(z_pos)
  [b_hallA] -> F01_01_Edge_Detector/1(b_hallA)
  F01_01_Edge_Detector/1("b_edge ") -> [b_edge]
  F01_03_Direction_Detection/1(z_dir) -> [z_dir]
  [b_hallB] -> F01_01_Edge_Detector/2(b_hallB)
  [b_hallC] -> F01_01_Edge_Detector/3(b_hallC)
  b_hallA/1 -> [b_hallA]
  b_hallB/1 -> [b_hallB]
  b_hallC/1 -> [b_hallC]
  [b_hallC] -> F01_02_Position_Calculation/3(b_hallC)
  [b_hallB] -> F01_02_Position_Calculation/2(b_hallB)
  [b_hallA] -> F01_02_Position_Calculation/1(b_hallA)
  F01_02_Position_Calculation/2("z_pos ") -> [z_pos]
  [b_edge] -> F01_04_Speed_Estimation/1(b_edge)
  F01_04_Speed_Estimation/1(n_mot) -> [n_mot]
  [n_mot] -> "n_mot "/1
  [z_pos] -> z_pos/1
  [z_dir] -> F01_04_Speed_Estimation/2(z_dir)
  F01_04_Speed_Estimation/3(z_counter) -> [z_counter]
  F01_04_Speed_Estimation/4(z_counterRaw) -> [z_counterRaw]
  F01_03_Direction_Detection/2(z_dirPrev) -> [z_dirPrev]
  [z_dirPrev] -> F01_04_Speed_Estimation/3(z_dirPrev)
  [z_pos] -> F01_05_Electrical_Angle_Estimation/1(z_pos)
  [z_dir] -> F01_05_Electrical_Angle_Estimation/2(z_dir)
  [z_counter] -> F01_05_Electrical_Angle_Estimation/3(z_counter)
  [z_counterRaw] -> F01_05_Electrical_Angle_Estimation/4(z_counterRaw)
  [b_enaAdvCtrl] -> F01_05_Electrical_Angle_Estimation/5(b_enaAdvCtrl)
  F01_04_Speed_Estimation/6(b_enaAdvCtrl) -> [b_enaAdvCtrl]
  [b_enaAdvCtrl] -> b_enaAdvCtrl/1
  [a_elecAngle] -> a_elecAngle/1
  F01_04_Speed_Estimation/2(n_motAbs) -> [n_motAbs]
  [n_motAbs] -> n_motAbs/1
  F01_02_Position_Calculation/1(z_posRaw) -> [z_posRaw]
  [z_posRaw] -> z_posRaw/1
  [b_motStdStill] -> b_motStdStill/1
  F01_04_Speed_Estimation/5(b_motStdStill) -> [b_motStdStill]
  [z_dir] -> z_dir/1
  a_encoderCNT/1 -> [a_encoderCNT]
  b_angleMeasEna/1 -> If1/1
  If1/1 -> F01_05_Electrical_Angle_Estimation/Action
  If1/2 -> F01_06_Electrical_Angle_Measurement/Action
  F01_05_Electrical_Angle_Estimation/1(a_elecAngle) -> Merge/1
  Merge/1 -> [a_elecAngle]
  F01_06_Electrical_Angle_Measurement/1(a_elecAngle) -> Merge/2
  [a_encoderCNT] -> F01_06_Electrical_Angle_Measurement/1(a_encoderCNT)
  a_mechangle/1 -> [a_mechangle]
  [a_mechangle] -> F01_06_Electrical_Angle_Measurement/2(a_mechangle)

== system BLDCmotor_FOC_R2017b_fixdt/BLDC_controller/F02_Diagnostics ==
  b_motEna : Inport
  z_posRaw : Inport  Port=2
  b_motStdStill : Inport  Port=3
  VqFinPrev : Inport  Port=4
  function : TriggerPort  TriggerType=function-call  VariantControl=Variant
  Diagnostics_Enabled : Subsystem
  If2 : If  IfExpression=u1 ~= 0  ShowElse=off
  b_diagEna : Constant  Value=b_diagEna  OutDataTypeStr=boolean
  "z_errCode " : Outport  InitialOutput=0  VectorParamsAs1DForOutWhenUnconnected=off
  b_errFlag : Outport  Port=2  InitialOutput=0  VectorParamsAs1DForOutWhenUnconnected=off
  wires:
  [z_errCode] -> "z_errCode "/1
  z_posRaw/1 -> [z_posRaw]
  Diagnostics_Enabled/2(b_errFlag) -> [b_errFlag]
  [b_errFlag] -> b_errFlag/1
  VqFinPrev/1 -> [VqFinPrev]
  b_motStdStill/1 -> [b_motStdStill]
  b_motEna/1 -> [b_motEna]
  b_diagEna/1 -> If2/1
  [VqFinPrev] -> Diagnostics_Enabled/4(VqFinPrev)
  Diagnostics_Enabled/1("z_errCode ") -> [z_errCode]
  [b_motStdStill] -> Diagnostics_Enabled/3(b_motStdStill)
  [b_motEna] -> Diagnostics_Enabled/1(b_motEna)
  [z_posRaw] -> Diagnostics_Enabled/2(z_posRaw)
  If2/1 -> Diagnostics_Enabled/Action

== system BLDCmotor_FOC_R2017b_fixdt/BLDC_controller/F03_Control_Mode_Manager ==
  b_errFlag : Inport
  b_motEna : Inport  Port=2
  b_cruiseCtrlEna : Inport  Port=3
  z_ctrlTypSel : Inport  Port=4
  z_ctrlModReq : Inport  Port=5
  r_inpTgt : Inport  Port=6
  VqFinPrev : Inport  Port=7
  function : TriggerPort  TriggerType=function-call  VariantControl=Variant
  Abs1 : Abs  OutDataTypeStr=Inherit: Inherit via back propagation  RndMeth=Zero  SaturateOnIntegerOverflow=off
  F03_01_Mode_Transition_Calculation : Subsystem
  F03_02_Control_Mode_Manager : Stateflow chart  TreatAsAtomicUnit=on
  F03_03_Input_Target_Synthesis : Subsystem
  z_ctrlMod : Outport  VectorParamsAs1DForOutWhenUnconnected=off
  r_inpTgtScaAbs : Outport  Port=2  VectorParamsAs1DForOutWhenUnconnected=off
  r_inpTgtSca : Outport  Port=3  VectorParamsAs1DForOutWhenUnconnected=off
  r_inpTgtConv : Outport  Port=4  OutputWhenDisabled=reset  InitialOutput=0  VectorParamsAs1DForOutWhenUnconnected=off
  wires:
  [z_ctrlMod] -> z_ctrlMod/1
  b_motEna/1 -> [b_motEna]
  [b_toOpen] -> F03_02_Control_Mode_Manager/1(b_toOpen)
  [b_toSpdMod] -> F03_02_Control_Mode_Manager/3(b_toSpdMod)
  z_ctrlModReq/1 -> [z_ctrlModReq]
  [b_toTrqMod] -> F03_02_Control_Mode_Manager/4(b_toTrqMod)
  F03_02_Control_Mode_Manager/1(z_ctrlMod) -> [z_ctrlMod]
  [b_toActive] -> F03_02_Control_Mode_Manager/2(b_toActive)
  F03_01_Mode_Transition_Calculation/1(b_toOpen) -> [b_toOpen]
  F03_01_Mode_Transition_Calculation/2(b_toActive) -> [b_toActive]
  F03_01_Mode_Transition_Calculation/3(b_toSpdMod) -> [b_toSpdMod]
  F03_01_Mode_Transition_Calculation/4(b_toTrqMod) -> [b_toTrqMod]
  [b_motEna] -> F03_01_Mode_Transition_Calculation/2(b_motEna)
  [z_ctrlModReq] -> F03_01_Mode_Transition_Calculation/4(z_ctrlModReq)
  b_errFlag/1 -> [b_errFlag]
  [b_errFlag] -> F03_01_Mode_Transition_Calculation/1(b_errFlag)
  [z_ctrlModReq] -> F03_03_Input_Target_Synthesis/2(z_ctrlModReq)
  [z_ctrlTypSel] -> F03_03_Input_Target_Synthesis/1(z_ctrlTypSel)
  [r_inpTgt] -> F03_03_Input_Target_Synthesis/4(r_inpTgt)
  F03_03_Input_Target_Synthesis/1(r_inpTgtSca) -> Abs1/1, [r_inpTgtSca]
  [z_ctrlMod] -> F03_03_Input_Target_Synthesis/3(z_ctrlMod)
  VqFinPrev/1 -> [VqFinPrev]
  [VqFinPrev] -> F03_03_Input_Target_Synthesis/5(VqFinPrev)
  r_inpTgt/1 -> [r_inpTgt]
  z_ctrlTypSel/1 -> [z_ctrlTypSel]
  [r_inpTgtSca] -> r_inpTgtSca/1
  b_cruiseCtrlEna/1 -> [b_cruiseCtrlEna]
  [b_cruiseCtrlEna] -> F03_01_Mode_Transition_Calculation/3(b_cruiseCtrlEna)
  Abs1/1 -> [r_inpTgtScaAbs]
  [r_inpTgtScaAbs] -> r_inpTgtScaAbs/1
  F03_03_Input_Target_Synthesis/2(r_inpTgtConv) -> [r_inpTgtConv]
  [r_inpTgtConv] -> r_inpTgtConv/1

== system BLDCmotor_FOC_R2017b_fixdt/BLDC_controller/F04_Field_Weakening ==
  z_ctrlTypSel : Inport
  r_inpTgtConv : Inport  Port=2
  n_motAbs : Inport  Port=3
  function : TriggerPort  TriggerType=function-call  VariantControl=Variant
  FieldWeakening : Scope  NumInputPorts=3
      settings: ActiveDisplayYMinimum=-253.96212325882078  ActiveDisplayYMaximum=924.69141656240208  DataLoggingVariableName=ScopeData9
  Field_Weakening_Enabled : Subsystem
  If3 : If  IfExpression=u1 ~= 0  ShowElse=off
  b_fieldWeakEna : Constant  Value=b_fieldWeakEna  OutDataTypeStr=boolean
  "r_fieldWeak " : Outport  InitialOutput=0  VectorParamsAs1DForOutWhenUnconnected=off
  wires:
  [r_fieldWeak] -> "r_fieldWeak "/1
  n_motAbs/1 -> [n_motAbs]
  r_inpTgtConv/1 -> [r_inpTgtConv]
  If3/1 -> Field_Weakening_Enabled/Action
  [n_motAbs] -> FieldWeakening/2, Field_Weakening_Enabled/3(n_motAbs)
  [r_inpTgtConv] -> FieldWeakening/3, Field_Weakening_Enabled/2(r_inpTgtConv)
  [z_ctrlTypSel] -> Field_Weakening_Enabled/1(z_ctrlTypSel)
  Field_Weakening_Enabled/1("r_fieldWeak ") -> FieldWeakening/1, [r_fieldWeak]
  b_fieldWeakEna/1 -> If3/1
  z_ctrlTypSel/1 -> [z_ctrlTypSel]

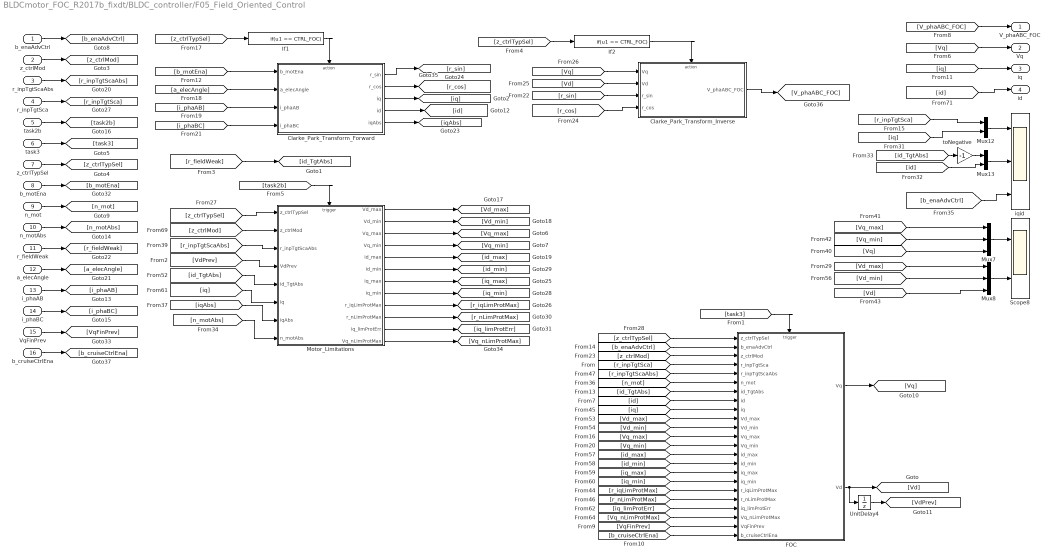
== system BLDCmotor_FOC_R2017b_fixdt/BLDC_controller/F05_Field_Oriented_Control ==
  b_enaAdvCtrl : Inport
  z_ctrlMod : Inport  Port=2
  r_inpTgtScaAbs : Inport  Port=3
  r_inpTgtSca : Inport  Port=4
  task2b : Inport  Port=5
  task3 : Inport  Port=6
  z_ctrlTypSel : Inport  Port=7
  b_motEna : Inport  Port=8
  n_mot : Inport  Port=9
  n_motAbs : Inport  Port=10
  r_fieldWeak : Inport  Port=11
  a_elecAngle : Inport  Port=12
  i_phaAB : Inport  Port=13
  i_phaBC : Inport  Port=14
  VqFinPrev : Inport  Port=15
  b_cruiseCtrlEna : Inport  Port=16
  Clarke_Park_Transform_Forward : Subsystem
  Clarke_Park_Transform_Inverse : Subsystem
  FOC : Subsystem
  If1 : If  IfExpression=u1 == CTRL_FOC  ShowElse=off
  If2 : If  IfExpression=u1 == CTRL_FOC  ShowElse=off
  Motor_Limitations : Subsystem
  Mux12 : Mux  Inputs=2
  Mux13 : Mux  Inputs=2
  Mux7 : Mux  Inputs=3
  Mux8 : Mux  Inputs=3
  Scope8 : Scope  NumInputPorts=2
      settings: ActiveDisplayYMinimum=-648.22605304081912  ActiveDisplayYMaximum=4217.88501843494
  UnitDelay4 : UnitDelay  SampleTime=-1  HasFrameUpgradeWarning=on
      settings: AttributesFormatString=Ini=%<X0>
  iqid : Scope  NumInputPorts=3
      settings: ActiveDisplayYMinimum=7.4520959693970212  ActiveDisplayYMaximum=508.73162154068666  DataLoggingVariableName=ScopeData11
  toNegative : Gain  Tag=struct('comment',struct('text','','placement',1),'logdata',struct('maxnumvals',inf,'plotchannels',[],'loggingmode',3,'channels',1),'output',struct('variable','','description','','name','$S_$B','width',1,'address','','max',NaN,'min',NaN,'class','default','type','CONTINUOUS','scaling','','lsb',1,'offset',0,'arb',0,'freeze',1,'unit','','autoscalingmode',1,'lowerheadroom',1,'upperheadroom',1,'headroomunit','bit','keepdatatype',1,'checkmin',0,'checkmax',0,'castoutput',0,'show',0),'gain',struct('variable','','description','','name','$S_$B_gain','width',1,'address','','max',NaN,'min',NaN,'class','default','type','CONTINUOUS','scaling','','lsb',1,'offset',0,'arb',0,'freeze',1,'unit','','keepdatatype',1,'value','1','scalar',0,'tolerance',1),'scalingvalid',0,'date',730486)  Gain=-1  RndMeth=Zero  OutDataTypeStr=Inherit: Same as input  ParamDataTypeStr=Inherit: Same as input
  V_phaABC_FOC : Outport  OutputWhenDisabled=reset  InitialOutput=0  VectorParamsAs1DForOutWhenUnconnected=off
  Vq : Outport  Port=2  VectorParamsAs1DForOutWhenUnconnected=off
  iq : Outport  Port=3  OutputWhenDisabled=reset  InitialOutput=0  VectorParamsAs1DForOutWhenUnconnected=off
  id : Outport  Port=4  OutputWhenDisabled=reset  InitialOutput=0  VectorParamsAs1DForOutWhenUnconnected=off
  wires:
  [V_phaABC_FOC] -> V_phaABC_FOC/1
  i_phaAB/1 -> [i_phaAB]
  i_phaBC/1 -> [i_phaBC]
  Mux12/1 -> iqid/1
  Mux13/1 -> iqid/2
  [r_inpTgtSca] -> Mux12/1
  [iq] -> Mux12/2
  [id] -> Mux13/2
  [id_TgtAbs] -> toNegative/1
  r_inpTgtSca/1 -> [r_inpTgtSca]
  [Vd_max] -> Mux8/1
  [Vd] -> Mux8/3
  Mux8/1 -> Scope8/2
  [Vd_min] -> Mux8/2
  Mux7/1 -> Scope8/1
  [Vq_min] -> Mux7/2
  [Vq] -> Vq/1
  b_enaAdvCtrl/1 -> [b_enaAdvCtrl]
  z_ctrlMod/1 -> [z_ctrlMod]
  n_mot/1 -> [n_mot]
  [b_enaAdvCtrl] -> iqid/3
  Motor_Limitations/3(Vq_max) -> [Vq_max]
  Motor_Limitations/4(Vq_min) -> [Vq_min]
  [VdPrev] -> Motor_Limitations/4(VdPrev)
  [id_TgtAbs] -> Motor_Limitations/5(id_TgtAbs)
  Motor_Limitations/2(Vd_min) -> [Vd_min]
  Motor_Limitations/1(Vd_max) -> [Vd_max]
  Motor_Limitations/5(id_max) -> [id_max]
  Motor_Limitations/6(id_min) -> [id_min]
  Motor_Limitations/7(iq_max) -> [iq_max]
  Motor_Limitations/8(iq_min) -> [iq_min]
  [iq] -> Motor_Limitations/6(iq)
  Motor_Limitations/11(iq_limProtErr) -> [iq_limProtErr]
  Motor_Limitations/12(Vq_nLimProtMax) -> [Vq_nLimProtMax]
  [z_ctrlMod] -> Motor_Limitations/2(z_ctrlMod)
  r_fieldWeak/1 -> [r_fieldWeak]
  a_elecAngle/1 -> [a_elecAngle]
  [id] -> id/1
  [iq] -> iq/1
  b_motEna/1 -> [b_motEna]
  task2b/1 -> [task2b]
  task3/1 -> [task3]
  FOC/1(Vq) -> [Vq]
  [b_enaAdvCtrl] -> FOC/2(b_enaAdvCtrl)
  [id_TgtAbs] -> FOC/7(id_TgtAbs)
  [id] -> FOC/8(id)
  [Vd_max] -> FOC/10(Vd_max)
  [Vd_min] -> FOC/11(Vd_min)
  [id_max] -> FOC/14(id_max)
  [id_min] -> FOC/15(id_min)
  [r_inpTgtSca] -> FOC/4(r_inpTgtSca)
  [Vq_max] -> FOC/12(Vq_max)
  [Vq_min] -> FOC/13(Vq_min)
  [iq_limProtErr] -> FOC/20(iq_limProtErr)
  [Vq_nLimProtMax] -> FOC/21(Vq_nLimProtMax)
  [iq_max] -> FOC/16(iq_max)
  [iq_min] -> FOC/17(iq_min)
  [iq] -> FOC/9(iq)
  [n_mot] -> FOC/6(n_mot)
  [z_ctrlMod] -> FOC/3(z_ctrlMod)
  FOC/2(Vd) -> UnitDelay4/1, [Vd]
  UnitDelay4/1 -> [VdPrev]
  n_motAbs/1 -> [n_motAbs]
  [n_motAbs] -> Motor_Limitations/8(n_motAbs)
  [iqAbs] -> Motor_Limitations/7(iqAbs)
  [r_inpTgtScaAbs] -> Motor_Limitations/3(r_inpTgtScaAbs)
  Motor_Limitations/9(r_iqLimProtMax) -> [r_iqLimProtMax]
  [r_iqLimProtMax] -> FOC/18(r_iqLimProtMax)
  Motor_Limitations/10(r_nLimProtMax) -> [r_nLimProtMax]
  [r_nLimProtMax] -> FOC/19(r_nLimProtMax)
  [r_inpTgtScaAbs] -> FOC/5(r_inpTgtScaAbs)
  VqFinPrev/1 -> [VqFinPrev]
  [VqFinPrev] -> FOC/22(VqFinPrev)
  [b_cruiseCtrlEna] -> FOC/23(b_cruiseCtrlEna)
  b_cruiseCtrlEna/1 -> [b_cruiseCtrlEna]
  [task2b] -> Motor_Limitations/Trigger
  [task3] -> FOC/Trigger
  r_inpTgtScaAbs/1 -> [r_inpTgtScaAbs]
  toNegative/1 -> Mux13/1
  If1/1 -> Clarke_Park_Transform_Forward/Action
  [r_fieldWeak] -> [id_TgtAbs]
  [b_motEna] -> Clarke_Park_Transform_Forward/1(b_motEna)
  [a_elecAngle] -> Clarke_Park_Transform_Forward/2(a_elecAngle)
  [i_phaAB] -> Clarke_Park_Transform_Forward/3(i_phaAB)
  [i_phaBC] -> Clarke_Park_Transform_Forward/4(i_phaBC)
  Clarke_Park_Transform_Forward/3(iq) -> [iq]
  Clarke_Park_Transform_Forward/4(id) -> [id]
  Clarke_Park_Transform_Forward/5(iqAbs) -> [iqAbs]
  Clarke_Park_Transform_Forward/1(r_sin) -> [r_sin]
  Clarke_Park_Transform_Forward/2(r_cos) -> [r_cos]
  [Vq] -> Clarke_Park_Transform_Inverse/1(Vq)
  [Vd] -> Clarke_Park_Transform_Inverse/2(Vd)
  [r_sin] -> Clarke_Park_Transform_Inverse/3(r_sin)
  [r_cos] -> Clarke_Park_Transform_Inverse/4(r_cos)
  Clarke_Park_Transform_Inverse/1(V_phaABC_FOC) -> [V_phaABC_FOC]
  If2/1 -> Clarke_Park_Transform_Inverse/Action
  z_ctrlTypSel/1 -> [z_ctrlTypSel]
  [z_ctrlTypSel] -> If1/1
  [z_ctrlTypSel] -> If2/1
  [z_ctrlTypSel] -> Motor_Limitations/1(z_ctrlTypSel)
  [z_ctrlTypSel] -> FOC/1(z_ctrlTypSel)
  [Vq] -> Mux7/3
  [Vq_max] -> Mux7/1

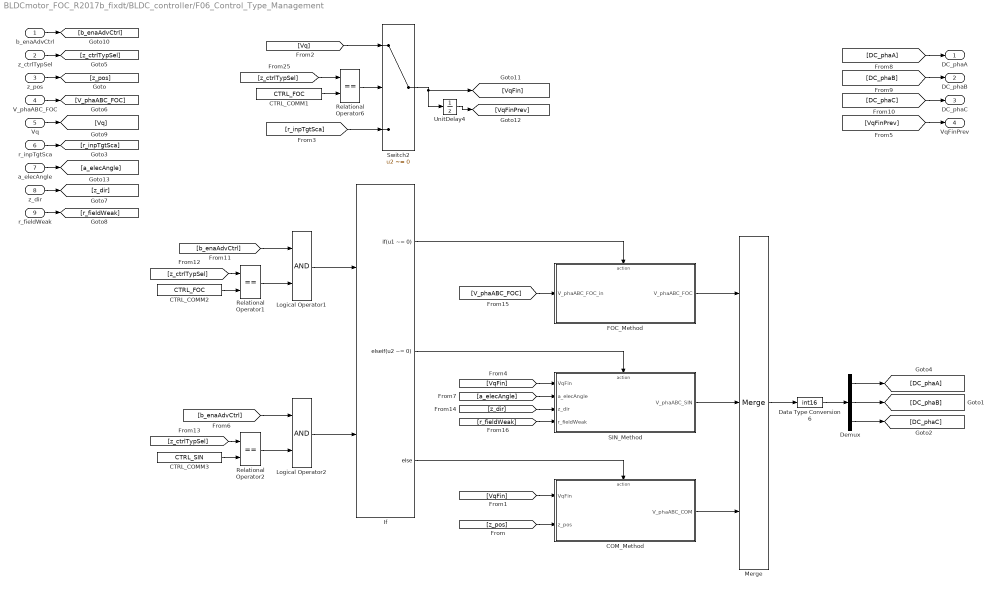
== system BLDCmotor_FOC_R2017b_fixdt/BLDC_controller/F06_Control_Type_Management ==
  b_enaAdvCtrl : Inport
  z_ctrlTypSel : Inport  Port=2
  z_pos : Inport  Port=3
  V_phaABC_FOC : Inport  Port=4
  Vq : Inport  Port=5
  r_inpTgtSca : Inport  Port=6
  a_elecAngle : Inport  Port=7
  z_dir : Inport  Port=8
  r_fieldWeak : Inport  Port=9
  COM_Method : Subsystem
  CTRL_COMM1 : Constant  Value=CTRL_FOC  OutDataTypeStr=Inherit: Inherit via back propagation
  CTRL_COMM2 : Constant  Value=CTRL_FOC  OutDataTypeStr=Inherit: Inherit via back propagation
  CTRL_COMM3 : Constant  Value=CTRL_SIN  OutDataTypeStr=Inherit: Inherit via back propagation
  Data Type Conversion6 : DataTypeConversion  OutDataTypeStr=int16  SaturateOnIntegerOverflow=off  RndMeth=Floor
  Demux : Demux  Outputs=3
  FOC_Method : Subsystem
  If : If  NumInputs=2  IfExpression=u1 ~= 0  ElseIfExpressions=u2 ~= 0
  Logical Operator1 : Logic  AllPortsSameDT=off  OutDataTypeStr=boolean
  Logical Operator2 : Logic  AllPortsSameDT=off  OutDataTypeStr=boolean
  Merge : Merge  Inputs=3
  Relational Operator1 : RelationalOperator  Operator===  OutDataTypeStr=boolean  RndMeth=Simplest  InputSameDT=off
  Relational Operator2 : RelationalOperator  Operator===  OutDataTypeStr=boolean  RndMeth=Simplest  InputSameDT=off
  Relational Operator6 : RelationalOperator  Operator===  OutDataTypeStr=boolean  RndMeth=Simplest  InputSameDT=off
  SIN_Method : Subsystem
  Switch2 : Switch  Criteria=u2 ~= 0  OutDataTypeStr=Inherit: Inherit via back propagation  RndMeth=Zero  SaturateOnIntegerOverflow=off  InputSameDT=off
  UnitDelay4 : UnitDelay  SampleTime=-1  HasFrameUpgradeWarning=on
      settings: AttributesFormatString=Ini=%<X0>
  DC_phaA : Outport  OutputWhenDisabled=reset  InitialOutput=0  VectorParamsAs1DForOutWhenUnconnected=off
  DC_phaB : Outport  Port=2  OutputWhenDisabled=reset  InitialOutput=0  VectorParamsAs1DForOutWhenUnconnected=off
  "DC_phaC " : Outport  Port=3  OutputWhenDisabled=reset  InitialOutput=0  VectorParamsAs1DForOutWhenUnconnected=off
  VqFinPrev : Outport  Port=4  OutputWhenDisabled=reset  InitialOutput=0  VectorParamsAs1DForOutWhenUnconnected=off
  wires:
  Demux/3 -> [DC_phaC]
  Demux/2 -> [DC_phaB]
  Demux/1 -> [DC_phaA]
  z_pos/1 -> [z_pos]
  [DC_phaC] -> "DC_phaC "/1
  [DC_phaB] -> DC_phaB/1
  [DC_phaA] -> DC_phaA/1
  Merge/1 -> Data Type Conversion6/1
  V_phaABC_FOC/1 -> [V_phaABC_FOC]
  Vq/1 -> [Vq]
  b_enaAdvCtrl/1 -> [b_enaAdvCtrl]
  [z_ctrlTypSel] -> Relational Operator6/1
  CTRL_COMM1/1 -> Relational Operator6/2
  Relational Operator6/1 -> Switch2/2
  r_inpTgtSca/1 -> [r_inpTgtSca]
  z_ctrlTypSel/1 -> [z_ctrlTypSel]
  Switch2/1 -> UnitDelay4/1, [VqFin]
  UnitDelay4/1 -> [VqFinPrev]
  [VqFinPrev] -> VqFinPrev/1
  [Vq] -> Switch2/1
  [r_inpTgtSca] -> Switch2/3
  Data Type Conversion6/1 -> Demux/1
  CTRL_COMM2/1 -> Relational Operator1/2
  [z_ctrlTypSel] -> Relational Operator1/1
  Relational Operator1/1 -> Logical Operator1/2
  [b_enaAdvCtrl] -> Logical Operator1/1
  [z_ctrlTypSel] -> Relational Operator2/1
  CTRL_COMM3/1 -> Relational Operator2/2
  [V_phaABC_FOC] -> FOC_Method/1(V_phaABC_FOC_in)
  If/3 -> COM_Method/Action
  COM_Method/1(V_phaABC_COM) -> Merge/3
  [z_pos] -> COM_Method/2(z_pos)
  [VqFin] -> COM_Method/1(VqFin)
  [VqFin] -> SIN_Method/1(VqFin)
  Logical Operator1/1 -> If/1
  If/2 -> SIN_Method/Action
  SIN_Method/1(V_phaABC_SIN) -> Merge/2
  FOC_Method/1(V_phaABC_FOC) -> Merge/1
  If/1 -> FOC_Method/Action
  Relational Operator2/1 -> Logical Operator2/2
  Logical Operator2/1 -> If/2
  [b_enaAdvCtrl] -> Logical Operator2/1
  a_elecAngle/1 -> [a_elecAngle]
  z_dir/1 -> [z_dir]
  r_fieldWeak/1 -> [r_fieldWeak]
  [a_elecAngle] -> SIN_Method/2(a_elecAngle)
  [z_dir] -> SIN_Method/3(z_dir)
  [r_fieldWeak] -> SIN_Method/4(r_fieldWeak)

== system BLDCmotor_FOC_R2017b_fixdt/BLDC_controller/Implemented_control_methods ==

== system BLDCmotor_FOC_R2017b_fixdt/BLDC_model_closed/__InputSSForSFun__ ==
  gates_PWM : Inport
  Tm_Nm : Inport  Port=2
  __UniqueOutportName__1__ : Outport  VectorParamsAs1DForOutWhenUnconnected=off
  __UniqueOutportName__2__ : Outport  Port=2  VectorParamsAs1DForOutWhenUnconnected=off
  wires:
  gates_PWM/1 -> __UniqueOutportName__1__/1
  Tm_Nm/1 -> __UniqueOutportName__2__/1
